simulink model "DCDC_4PHASE"  (R2022b)
settings: Solver=ode45  StartTime=0.0  StopTime=1  RelTol=1e-3  EnableMultiTasking=on
undefined symbols (not defined in the file): Acid, Lead
libraries: spsSeriesRLCBranchLib x21, spsIGBTDiodeLib x9, spsVoltageMeasurementLib x3, spsBatteryLib x1, spsCurrentMeasurementLib x1, spsDiodeLib x1, spsIdealSwitchLib x1, spsDCVoltageSourceLib x1, spspowerguiLib x1
settings Model: SimulationMode=accelerator  Creator=ZTE  LastModifiedBy=Drawing Sword
settings SolverCC: AlgebraicLoopSolver=TrustRegion
settings DataIOCC: LimitDataPoints=on  SaveFormat=Array  SignalLoggingSaveFormat=ModelDataLogs  ReturnWorkspaceOutputs=off
settings OptimizationCC: ExpressionDepthLimit=2147483647  LifeSpan=inf
settings DebuggingCC: UnderspecifiedInitializationDetection=Classic  MergeDetectMultiDrivingBlocksExec=none  FcnCallInpInsideContextMsg=warning  UnconnectedInputMsg=warning  UnconnectedOutputMsg=warning  UnconnectedLineMsg=warning  AllowSymbolicDim=off  StateNameClashWarn=warning  SFUnexpectedBacktrackingDiag=warning  SFNoUnconditionalDefaultTransitionDiag=warning  SFExecutionAtInitializationDiag=none  SFMachineParentedDataDiag=warning  ArithmeticOperatorsInVariantConditions=warning
settings HardwareCC: ProdBitPerPointer=32  ProdBitPerSizeT=32  ProdBitPerPtrDiffT=32  ProdLargestAtomicFloat=None  ProdIntDivRoundTo=Undefined  ProdEndianess=Unspecified  ProdWordSize=32  ProdHWDeviceType=32-bit Generic
settings ModelReferenceCC: EnableRefExpFcnMdlSchedulingChecks=on  PropagateSignalLabelsOutOfModel=off
settings SFSimCC: SimUseLocalCustomCode=off  CustomCodeUndefinedFunction=UseInterfaceOnly
settings RTWCC: RTWUseLocalCustomCode=off
settings CodeAppCC: StateflowObjectComments=on
settings GRTTargetCC: TargetLangStandard=C89/C90 (ANSI)  CombineOutputUpdateFcns=off  GRTInterface=on
settings ConfigComp: CovMetricSettings=dw  CovSaveCumulativeToWorkspaceVar=on  CovSaveSingleToWorkspaceVar=on  CovExternalEMLEnable=off
settings SimscapeCC: SimscapeNormalizeSystem=off

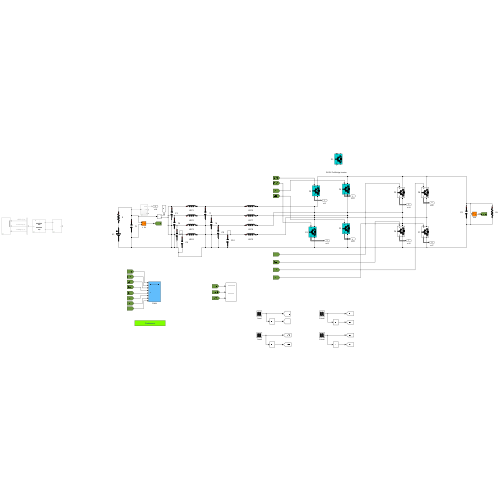
[thumbnail: Simulink's stored preview of the top-level diagram]
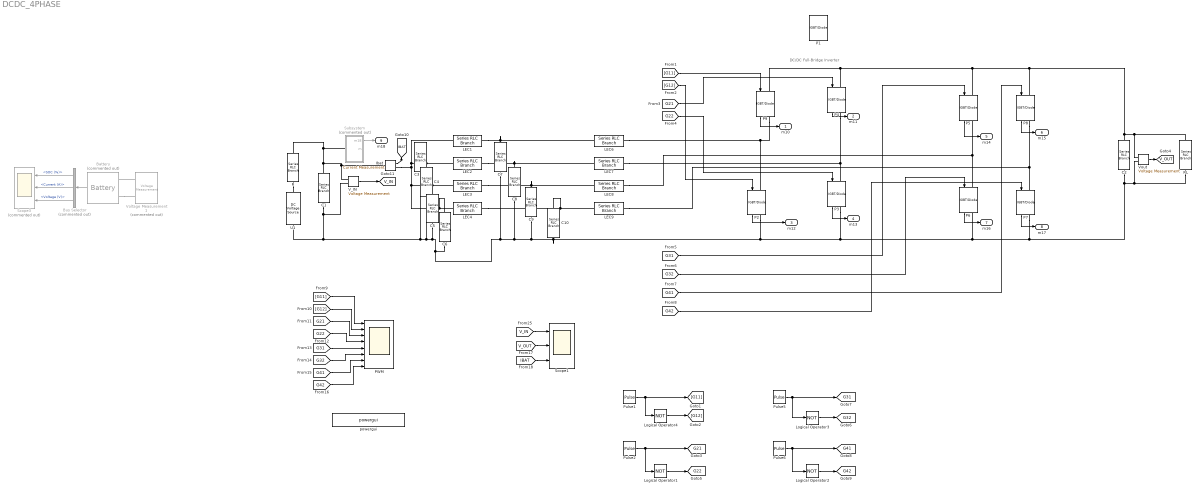
== system DCDC_4PHASE ==
  note: DC/DC Full-Bridge Inverter
  Battery : spsBatteryLib/Battery  Commented=on  BatType=Lead-Acid  ShowTempParam=off  ThermalPreset=no  ShowAgeParam=off  NomV=200  NomQ=5  SOC=80  Batt_Tr=30  PresetModel=on  MaxQ=5.2083  MinV=150  FullV=217.7632  Dis_rate=1  R=0.4  Normal_OP=1.5514  expZone="[203.6184    0.01666667]"  current=[6.5 13 32.5]  Units=Time  Tci=20  NomT=25  T2=0  MaxQ2=2.208  FullV2=3.45  Normal_OP2=2.8  expZone2="[3.22        0.23]"  Rca=0.6  ti=1000  Dp=0  Neq0=0  Tsim=1e6  Ta1=25  Qeol=5.4*0.9  Reol=0.013333*1.2  Char_age=[2.3478, 3]  Dis_age=[2.3478, 10]  N1=1500  N2=10500  N3=1000  N4=1400  Ta2=45  N5=950
  Bus Selector : BusSelector  Commented=on  OutputSignals=SOC (%),Current (A),Voltage (V)
  C1 : spsSeriesRLCBranchLib/Series RLC Branch  LConnTagsString=__new0  RConnTagsString=__new0  BranchType=C  Resistance=1  Inductance=1e-3  SetiL0=off  InitialCurrent=0  Capacitance=0.35  Setx0=off  InitialVoltage=0  Measurements=None
  C{7..10} (4 alike) : spsSeriesRLCBranchLib/Series RLC Branch  LConnTagsString=__new0  RConnTagsString=__new0  BranchType=C  Resistance=1  Inductance=1e-3  SetiL0=off  InitialCurrent=0  Capacitance=0.02  Setx0=off  InitialVoltage=0  Measurements=None
  C2 : spsSeriesRLCBranchLib/Series RLC Branch  LConnTagsString=__new0  RConnTagsString=__new0  BranchType=C  Resistance=1  Inductance=1e-3  SetiL0=off  InitialCurrent=0  Capacitance=0.64  Setx0=off  InitialVoltage=0  Measurements=Branch voltage and current
  C{3..6} (4 alike) : spsSeriesRLCBranchLib/Series RLC Branch  LConnTagsString=__new0  RConnTagsString=__new0  BranchType=C  Resistance=1  Inductance=1e-3  SetiL0=off  InitialCurrent=0  Capacitance=0.002  Setx0=off  InitialVoltage=0  Measurements=None
  Ibat : spsCurrentMeasurementLib/Current Measurement  PhasorSimulation=off  OutputType=Complex  PSBequivalent=0
  LEC{1..4} (4 alike) : spsSeriesRLCBranchLib/Series RLC Branch  LConnTagsString=__new0  RConnTagsString=__new0  BranchType=L  Resistance=0  Inductance=1e-6  SetiL0=off  InitialCurrent=0  Capacitance=0  Setx0=off  InitialVoltage=0  Measurements=Branch voltage and current
  LEC{6..9} (4 alike) : spsSeriesRLCBranchLib/Series RLC Branch  LConnTagsString=__new0  RConnTagsString=__new0  BranchType=L  Resistance=0  Inductance=340e-6  SetiL0=off  InitialCurrent=0  Capacitance=0  Setx0=off  InitialVoltage=0  Measurements=Branch voltage and current
  Logical Operator{1..4} (4 alike) : Logic  Operator=NOT  Inputs=1  AllPortsSameDT=off  OutDataTypeStr=boolean
  P{1..9} (9 alike) : spsIGBTDiodeLib/IGBT//Diode  Ron=1e-3  Rs=1e5  Cs=inf  Measurements=on
  PWM : Scope  NumInputPorts=8
  Pulse1 : DiscretePulseGenerator  PulseType=Time based  Amplitude=15  Period=40e-6  PulseWidth=20
  Pulse2 : DiscretePulseGenerator  PulseType=Time based  Amplitude=0  Period=40e-6  PulseWidth=46  PhaseDelay=10e-6
  Pulse5 : DiscretePulseGenerator  PulseType=Time based  Amplitude=0  Period=40e-6  PulseWidth=46  PhaseDelay=20e-6
  Pulse6 : DiscretePulseGenerator  PulseType=Time based  Amplitude=0  Period=40e-6  PulseWidth=46  PhaseDelay=30e-6
  R : spsSeriesRLCBranchLib/Series RLC Branch  LConnTagsString=__new0  RConnTagsString=__new0  BranchType=R  Resistance=0.00001  Inductance=1e-3  SetiL0=off  InitialCurrent=0  Capacitance=1e-6  Setx0=off  InitialVoltage=0  Measurements=Branch voltage and current
  RL : spsSeriesRLCBranchLib/Series RLC Branch  LConnTagsString=__new0  RConnTagsString=__new0  BranchType=R  Resistance=0.05  Inductance=1e-3  SetiL0=off  InitialCurrent=0  Capacitance=1e-6  Setx0=off  InitialVoltage=0  Measurements=Branch voltage and current
  Scope1 : Scope  NumInputPorts=3
  Scope3 : Scope  Commented=on  NumInputPorts=3
  Subsystem : Subsystem  Commented=on
  U1 : spsDCVoltageSourceLib/DC Voltage Source  Amplitude=200  Measurements=Voltage
  V_IN : spsVoltageMeasurementLib/Voltage Measurement  Tag=PoWeRsYsTeMmEaSuReMeNt  PhasorSimulation=off  OutputType=Magnitude  PSBequivalent=0
  Voltage Measurement1 : spsVoltageMeasurementLib/Voltage Measurement  Commented=on  PhasorSimulation=off  OutputType=Complex  PSBequivalent=0
  Vout : spsVoltageMeasurementLib/Voltage Measurement  Tag=PoWeRsYsTeMmEaSuReMeNt  PhasorSimulation=off  OutputType=Magnitude  PSBequivalent=0
  powergui : spspowerguiLib/powergui  SimulationMode=Continuous  SampleTime=50e-6  frequency=60  Iterations=50  frequencyindice=0  Pbase=100e6  ErrMax=1e-4  UnitsV=kV  UnitsW=MW  buscounter=0  FunctionMessages=off  echomessages=off  EnableUseOfTLC=off  CurrentSourceSwitches=off  DisableSnubberDevices=off  DisableRonSwitches=off  DisableVfSwitches=off  DisplayEquations=off  AutomaticDiscreteSolvers=off  SolverType=Tustin/Backward Euler (TBE)  Interpol=off  ExternalGateDelay=off  methode=off  Ts=0  x0status=blocks  SPID=off  SwTol=0  HookPort=off  NonlinearTolerance=1e-4  nMaxIteration=100  ContinueOnMaxIteration=off  RestoreLinks=warning  ResistiveCurrentMeasurement=off  Frange=[0:2:500]  Ylog=off  Xlog=on  ShowGrid=off  save=off  variable=ZData  structure=sps1phPWM1_str  ZoomFFT=on  StartTime=0.1-2/60  cycles=2  DisplayStyle=1  fundamental=60  FreqAxis=off  MaxFrequency=5000  frequencyindicesteady=1  RmsSteady=1  display=off
  m10 : Outport
  m11 : Outport  Port=2
  m12 : Outport  Port=3
  m13 : Outport  Port=4
  m14 : Outport  Port=5
  m15 : Outport  Port=6
  m16 : Outport  Port=7
  m17 : Outport  Port=8
  m18 : Outport  Port=9
  tag scope: G21=global, G22=global, G31=global, G32=global, G41=global, G42=global, IBAT=global, V_IN=global, V_OUT=global
  wires:
  Vout/1 -> [V_OUT]
  [V_IN] -> Scope1/1
  Battery/1 -> Bus Selector/1
  Bus Selector/1 -> Scope3/1  "<SOC (%)>"
  Bus Selector/2 -> Scope3/2  "<Current (A)>"
  Bus Selector/3 -> Scope3/3  "<Voltage (V)>"
  [V_OUT] -> Scope1/2
  P6/1 -> m16/1
  P7/1 -> m17/1
  P3/1 -> m13/1
  P4/1 -> m11/1
  P8/1 -> m15/1
  [G41] -> P8/1
  P5/1 -> m14/1
  [G32] -> P6/1
  [G42] -> P7/1
  [G31] -> P5/1
  [G12] -> P2/1
  [G22] -> P3/1
  [G11] -> P9/1
  [G21] -> P4/1
  [G11] -> PWM/1
  [G12] -> PWM/2
  [G21] -> PWM/3
  [G22] -> PWM/4
  Pulse6/1 -> Logical Operator2/1, [G41]
  Pulse5/1 -> Logical Operator3/1, [G31]
  Pulse2/1 -> Logical Operator1/1, [G21]
  [IBAT] -> Scope1/3
  Ibat/1 -> [IBAT]
  V_IN/1 -> [V_IN]
  Logical Operator1/1 -> [G22]
  Logical Operator2/1 -> [G42]
  Logical Operator3/1 -> [G32]
  [G42] -> PWM/8
  [G32] -> PWM/6
  [G31] -> PWM/5
  [G41] -> PWM/7
  Subsystem/1(m18) -> m18/1
  Pulse1/1 -> Logical Operator4/1, [G11]
  P9/1 -> m10/1
  P2/1 -> m12/1
  Logical Operator4/1 -> [G12]
  connections:
  R/RConn1 -- U1/RConn1
  RL/LConn1 -- Vout/LConn1 -- C2/LConn1 -- P8/LConn1 -- P5/LConn1 -- P4/LConn1 -- P9/LConn1
  P7/RConn1 -- P3/RConn1 -- P2/RConn1 -- C10/RConn1 -- C9/RConn1 -- C8/RConn1 -- V_IN/LConn2 -- C1/RConn1 -- U1/LConn1 -- C3/RConn1 -- C4/RConn1 -- C5/RConn1 -- C6/RConn1 -- C7/RConn1 -- P6/RConn1 -- Vout/LConn2 -- RL/RConn1 -- C2/RConn1
  Battery/LConn2 -- Voltage Measurement1/LConn2
  Voltage Measurement1/LConn1 -- Battery/LConn1
  LEC1/LConn1 -- C4/LConn1 -- LEC2/LConn1 -- Ibat/RConn1 -- C5/LConn1 -- LEC3/LConn1 -- LEC4/LConn1 -- C6/LConn1
  LEC1/RConn1 -- C7/LConn1 -- LEC6/LConn1
  LEC4/RConn1 -- C10/LConn1 -- LEC9/LConn1
  LEC7/RConn1 -- P3/LConn1 -- P4/RConn1
  P6/LConn1 -- LEC8/RConn1 -- P5/RConn1
  R/LConn1 -- V_IN/LConn1 -- Ibat/LConn1 -- C1/LConn1 -- Subsystem/LConn1
  LEC6/RConn1 -- P2/LConn1 -- P9/RConn1
  LEC2/RConn1 -- C8/LConn1 -- LEC7/LConn1
  LEC3/RConn1 -- C9/LConn1 -- LEC8/LConn1
  LEC9/RConn1 -- P8/RConn1 -- P7/LConn1

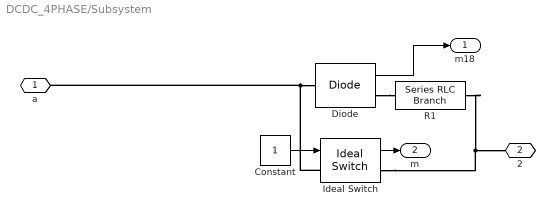
== system DCDC_4PHASE/Subsystem ==
  Constant : Constant
  Diode : spsDiodeLib/Diode  Ron=0.001  Lon=0  Vf=0.8  IC=0  UseSnubber=0  Rs=500  Cs=250e-9  Measurements=on
  Ideal Switch : spsIdealSwitchLib/Ideal Switch  Ron=0.001  Lon=0  IC=0  Rs=1e5  Cs=inf  Measurements=on
  R1 : spsSeriesRLCBranchLib/Series RLC Branch  LConnTagsString=__new0  RConnTagsString=__new0  BranchType=R  Resistance=0.1  Inductance=1e-3  SetiL0=off  InitialCurrent=0  Capacitance=1e-6  Setx0=off  InitialVoltage=0  Measurements=Branch voltage and current
  a : PMIOPort  Side=Left
  2 : PMIOPort  Port=2  Side=Right
  m18 : Outport
  m : Outport  Port=2
  wires:
  Constant/1 -> Ideal Switch/1
  Diode/1 -> m18/1
  Ideal Switch/1 -> m/1
  connections:
  Diode/RConn1 -- R1/RConn1
  Ideal Switch/LConn1 -- a/RConn1 -- Diode/LConn1
  R1/LConn1 -- 2/RConn1 -- Ideal Switch/RConn1
